simulink model "Part_2_Simulink"  (R2022b)
settings: Solver=VariableStepAuto  StartTime=0.0  StopTime=12  RelTol=1e-3
model workspace (MAT data in the model file):
  s = 351.26
  x = 425.72712
values from neighbouring files (symbols this model uses):
  Kd = PD.K    [Main.m]
  Kd_M = PD_M.K    [Main.m]
  Kd_O = PD_O.K    [Main.m]
  Kd_U = PD_U.K    [Main.m]
  Kp = -cell2mat(PD.Z)*Kd    [Main.m]
  Kp_M = -cell2mat(PD_M.Z)*Kd    [Main.m]
  Kp_O = -cell2mat(PD_O.Z)*Kd    [Main.m]
  Kp_U = -cell2mat(PD_U.Z)*Kd    [Main.m]
undefined symbols (not defined in the file or in its folder): sigbuilder_block
libraries: simulink_extras x10
settings Model: PacingRate=0.890000  Creator=AORUC19  LastModifiedBy=TANDAC20
settings OptimizationCC: ReuseModelBlockBuffer=on
settings DebuggingCC: UnconnectedInputMsg=warning  UnconnectedOutputMsg=warning  UnconnectedLineMsg=warning
settings ModelReferenceCC: EnableRefExpFcnMdlSchedulingChecks=on
settings RTWCC: DLArmComputeVersion=19.05

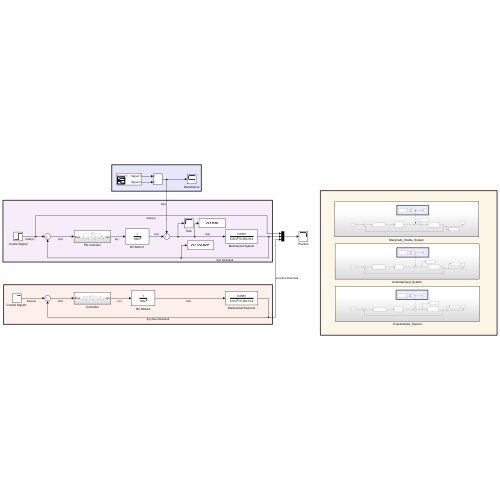
[thumbnail: Simulink's stored preview of the top-level diagram]
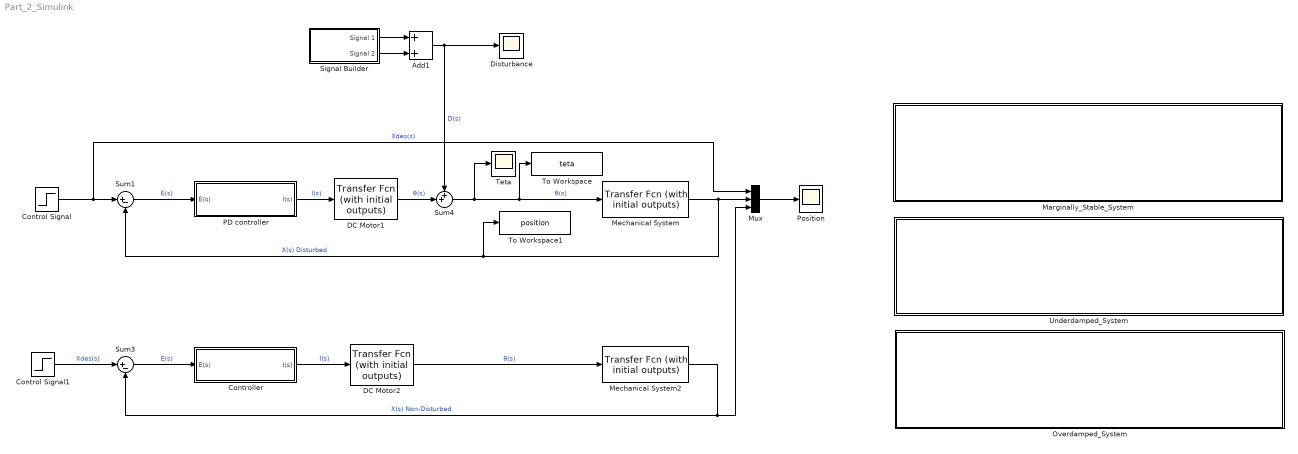
== system Part_2_Simulink ==
  Add1 : Sum
  Control Signal : Step  Time=0.3  Before=-1  After=0  SampleTime=0
  Control Signal1 : Step  Time=0.3  Before=-1  After=0  SampleTime=0
  Controller : Subsystem
  DC Motor1 : simulink_extras/Additional Linear/Transfer Fcn (with initial outputs)  N=[1]  D="[100  0 0]"  Y0=0  U0=0
  DC Motor2 : simulink_extras/Additional Linear/Transfer Fcn (with initial outputs)  N=[1]  D="[100  0 0]"  Y0=0  U0=0
  Disturbance : Scope
  Marginally_Stable_System : Subsystem
  Mechanical System : simulink_extras/Additional Linear/Transfer Fcn (with initial outputs)  N=[0.0981]  D="[0.01  0.05 0.2]"  Y0=0  U0=0
  Mechanical System2 : simulink_extras/Additional Linear/Transfer Fcn (with initial outputs)  N=[0.0981]  D="[0.01  0.05 0.2]"  Y0=0  U0=0
  Mux : Mux  Inputs=3
  Overdamped_System : Subsystem
  PD controller : Subsystem
  Position : Scope
  Signal Builder : Subsystem  Tag=STV Subsys  LoadFcn=sigbuilder_block('load');  StartFcn=sigbuilder_block('start');  StopFcn=sigbuilder_block('stop');  ClipboardFcn=sigbuilder_block('clipboard');  mask(Sigbuilder block){tuvar=[0:10]}
      mask help: Simulink:masks:SigbuilderBlock_MD
      mask init:
      | if ~strcmp(get_param(bdroot(gcbh),'SimulationStatus'),'stopped') tuvar = sigbuilder_block('maskInit'); end
      settings: CopyFcn=sigbuilder_block('copy');  DeleteFcn=sigbuilder_block('delete');  ModelCloseFcn=sigbuilder_block('modelClose');  PreSaveFcn=sigbuilder_block('preSave');  PauseFcn=sigbuilder_block('pause');  ContinueFcn=sigbuilder_block('continue');  NameChangeFcn=sigbuilder_block('namechange');  OpenFcn=sigbuilder_block('open',[437.6 199.2 550.4 400 ]);  CloseFcn=sigbuilder_block('close');
      mask Display: plot(0, 0, 100, 100,[2, 2, 32, 32, 2], [68, 8, 8, 68, 68],[32, 2], [38, 38], [32, 19, 2],[53, 60, 44], [32, 17, 17, 2],[16, 16, 31, 31]);txt = getActiveGroup(gcbh);text(2, 100, txt,'verticalAlignment', 'top');
  Sum1 : Sum  Inputs=|+-
  Sum3 : Sum  Inputs=|+-
  Sum4 : Sum  Inputs=++|
  Teta : Scope
  To Workspace : ToWorkspace  VariableName=teta  SampleTime=0.01
      settings: Save2DSignal=2-D array (concatenate along first dimension)
  To Workspace1 : ToWorkspace  VariableName=position  SampleTime=0.01
      settings: Save2DSignal=2-D array (concatenate along first dimension)
  Underdamped_System : Subsystem
  wires:
  Control Signal/1 -> Mux/1, Sum1/1  "Xdes(s)"
  Add1/1 -> Disturbance/1, Sum4/1  "D(s)"
  Signal Builder/2(Signal 2) -> Add1/2
  Signal Builder/1(Signal 1) -> Add1/1
  Mechanical System/1 -> Mux/2, To Workspace1/1, Sum1/2  "X(s) Disturbed"
  Mux/1 -> Position/1
  DC Motor2/1 -> Mechanical System2/1  "θ(s)"
  Mechanical System2/1 -> Sum3/2, Mux/3  "X(s) Non-Disturbed"
  Control Signal1/1 -> Sum3/1  "Xdes(s)"
  DC Motor1/1 -> Sum4/2  "θ(s)"
  Sum4/1 -> Mechanical System/1, To Workspace/1, Teta/1  "θ(s)"
  Sum3/1 -> Controller/1(E(s))  "E(s)"
  Controller/1(I(s)) -> DC Motor2/1  "I(s)"
  Sum1/1 -> PD controller/1(E(s))  "E(s)"
  PD controller/1(I(s)) -> DC Motor1/1  "I(s)"

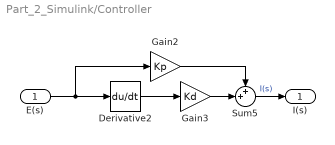
== system Part_2_Simulink/Controller ==
  E(s) : Inport
  Derivative2 : Derivative  CoefficientInTFapproximation=107.32
  Gain2 : Gain  Gain=Kp
  Gain3 : Gain  Gain=Kd
  Sum5 : Sum  Inputs=++|
  I(s) : Outport
  wires:
  Derivative2/1 -> Gain3/1
  E(s)/1 -> Derivative2/1, Gain2/1
  Gain3/1 -> Sum5/2
  Gain2/1 -> Sum5/1
  Sum5/1 -> I(s)/1  "I(s)"

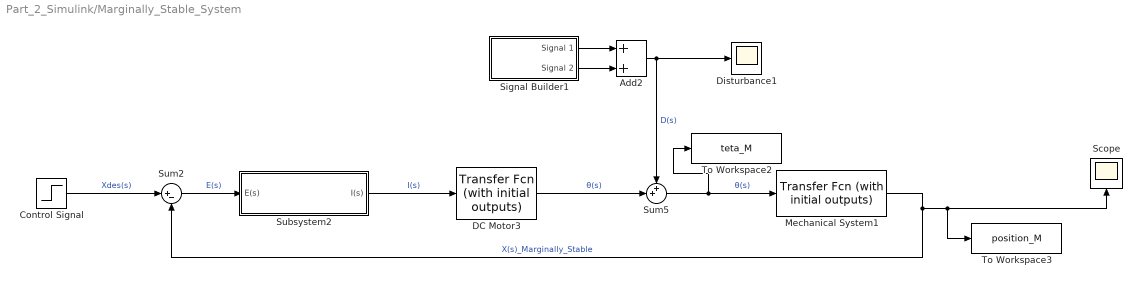
== system Part_2_Simulink/Marginally_Stable_System ==
  Add2 : Sum
  Control Signal : Step  Time=0  After=0  SampleTime=0
  DC Motor3 : simulink_extras/Additional Linear/Transfer Fcn (with initial outputs)  N=[1]  D="[100  0 0]"  Y0=0  U0=0
  Disturbance1 : Scope
  Mechanical System1 : simulink_extras/Additional Linear/Transfer Fcn (with initial outputs)  N=[0.0981]  D="[0.01  0.05 0.2]"  Y0=0  U0=0
  Scope : Scope
  Signal Builder1 : Subsystem  Tag=STV Subsys  LoadFcn=sigbuilder_block('load');  StartFcn=sigbuilder_block('start');  StopFcn=sigbuilder_block('stop');  ClipboardFcn=sigbuilder_block('clipboard');  mask(Sigbuilder block){tuvar=[0:10]}
      mask help: Simulink:masks:SigbuilderBlock_MD
      mask init:
      | if ~strcmp(get_param(bdroot(gcbh),'SimulationStatus'),'stopped') tuvar = sigbuilder_block('maskInit'); end
      settings: CopyFcn=sigbuilder_block('copy');  DeleteFcn=sigbuilder_block('delete');  ModelCloseFcn=sigbuilder_block('modelClose');  PreSaveFcn=sigbuilder_block('preSave');  PauseFcn=sigbuilder_block('pause');  ContinueFcn=sigbuilder_block('continue');  NameChangeFcn=sigbuilder_block('namechange');  OpenFcn=sigbuilder_block('open',[437.6 199.2 550.4 400 ]);  CloseFcn=sigbuilder_block('close');
      mask Display: plot(0, 0, 100, 100,[2, 2, 32, 32, 2], [68, 8, 8, 68, 68],[32, 2], [38, 38], [32, 19, 2],[53, 60, 44], [32, 17, 17, 2],[16, 16, 31, 31]);txt = getActiveGroup(gcbh);text(2, 100, txt,'verticalAlignment', 'top');
  Subsystem2 : Subsystem
  Sum2 : Sum  Inputs=|+-
  Sum5 : Sum  Inputs=++|
  To Workspace2 : ToWorkspace  VariableName=teta_M  SampleTime=0.01
      settings: Save2DSignal=2-D array (concatenate along first dimension)
  To Workspace3 : ToWorkspace  VariableName=position_M  SampleTime=0.01
      settings: Save2DSignal=2-D array (concatenate along first dimension)
  wires:
  Signal Builder1/1(Signal 1) -> Add2/1
  DC Motor3/1 -> Sum5/2  "θ(s)"
  Sum5/1 -> To Workspace2/1, Mechanical System1/1  "θ(s)"
  Signal Builder1/2(Signal 2) -> Add2/2
  Sum2/1 -> Subsystem2/1(E(s))  "E(s)"
  Mechanical System1/1 -> Scope/1, To Workspace3/1, Sum2/2  "X(s)_Marginally_Stable"
  Subsystem2/1(I(s)) -> DC Motor3/1  "I(s)"
  Add2/1 -> Disturbance1/1, Sum5/1  "D(s)"
  Control Signal/1 -> Sum2/1  "Xdes(s)"

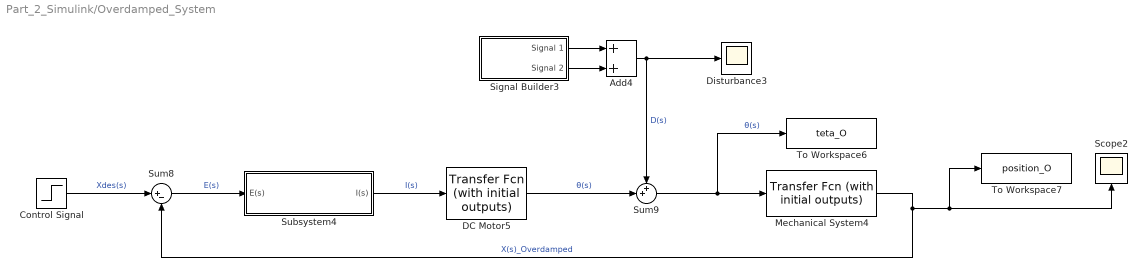
== system Part_2_Simulink/Overdamped_System ==
  Add4 : Sum
  Control Signal : Step  Time=0  After=0  SampleTime=0
  DC Motor5 : simulink_extras/Additional Linear/Transfer Fcn (with initial outputs)  N=[1]  D="[100  0 0]"  Y0=0  U0=0
  Disturbance3 : Scope
  Mechanical System4 : simulink_extras/Additional Linear/Transfer Fcn (with initial outputs)  N=[0.0981]  D="[0.01  0.05 0.2]"  Y0=0  U0=0
  Scope2 : Scope
  Signal Builder3 : Subsystem  Tag=STV Subsys  LoadFcn=sigbuilder_block('load');  StartFcn=sigbuilder_block('start');  StopFcn=sigbuilder_block('stop');  ClipboardFcn=sigbuilder_block('clipboard');  mask(Sigbuilder block){tuvar=[0:10]}
      mask help: Simulink:masks:SigbuilderBlock_MD
      mask init:
      | if ~strcmp(get_param(bdroot(gcbh),'SimulationStatus'),'stopped') tuvar = sigbuilder_block('maskInit'); end
      settings: CopyFcn=sigbuilder_block('copy');  DeleteFcn=sigbuilder_block('delete');  ModelCloseFcn=sigbuilder_block('modelClose');  PreSaveFcn=sigbuilder_block('preSave');  PauseFcn=sigbuilder_block('pause');  ContinueFcn=sigbuilder_block('continue');  NameChangeFcn=sigbuilder_block('namechange');  OpenFcn=sigbuilder_block('open',[437.6 199.2 550.4 400 ]);  CloseFcn=sigbuilder_block('close');
      mask Display: plot(0, 0, 100, 100,[2, 2, 32, 32, 2], [68, 8, 8, 68, 68],[32, 2], [38, 38], [32, 19, 2],[53, 60, 44], [32, 17, 17, 2],[16, 16, 31, 31]);txt = getActiveGroup(gcbh);text(2, 100, txt,'verticalAlignment', 'top');
  Subsystem4 : Subsystem
  Sum8 : Sum  Inputs=|+-
  Sum9 : Sum  Inputs=++|
  To Workspace6 : ToWorkspace  VariableName=teta_O  SampleTime=0.01
      settings: Save2DSignal=2-D array (concatenate along first dimension)
  To Workspace7 : ToWorkspace  VariableName=position_O  SampleTime=0.01
      settings: Save2DSignal=2-D array (concatenate along first dimension)
  wires:
  Add4/1 -> Disturbance3/1, Sum9/1  "D(s)"
  Signal Builder3/2(Signal 2) -> Add4/2
  Sum8/1 -> Subsystem4/1(E(s))  "E(s)"
  Mechanical System4/1 -> To Workspace7/1, Scope2/1, Sum8/2  "X(s)_Overdamped"
  Sum9/1 -> To Workspace6/1, Mechanical System4/1  "θ(s)"
  Signal Builder3/1(Signal 1) -> Add4/1
  DC Motor5/1 -> Sum9/2  "θ(s)"
  Subsystem4/1(I(s)) -> DC Motor5/1  "I(s)"
  Control Signal/1 -> Sum8/1  "Xdes(s)"

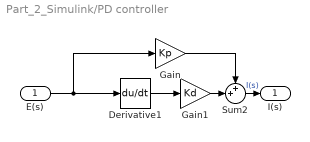
== system Part_2_Simulink/PD controller ==
  E(s) : Inport
  Derivative1 : Derivative  CoefficientInTFapproximation=107.32
  Gain : Gain  Gain=Kp
  Gain1 : Gain  Gain=Kd
  Sum2 : Sum  Inputs=++|
  I(s) : Outport
  wires:
  Gain/1 -> Sum2/1
  Derivative1/1 -> Gain1/1
  Gain1/1 -> Sum2/2
  Sum2/1 -> I(s)/1  "I(s)"
  E(s)/1 -> Gain/1, Derivative1/1

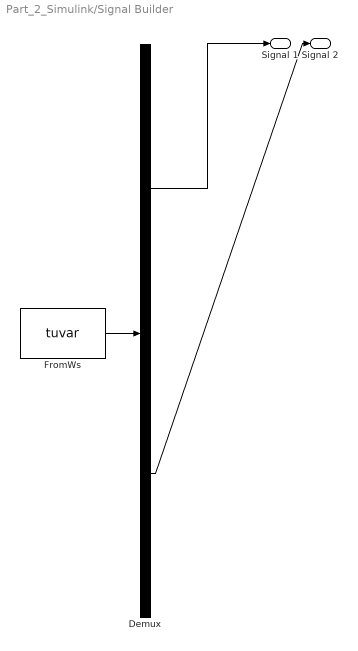
== system Part_2_Simulink/Signal Builder ==
  Demux : Demux  Tag=STV Demux  Outputs=2
      settings: DisplayOption=none
  FromWs : FromWorkspace  Tag=STV FromWs  VariableName=tuvar
      SigBuilderData=|
      | common.afterFinalStr = 'Extrapolate'
      | common.sampleTime = 0
      | dataSet.timeRange = [0 10]
      | dataSet.name = 'Group 1'
      | sbobj.Groups.Name = 'Group 1'
      | sbobj.Groups.Signals(1).Name = 'Signal 1'
      | sbobj.Groups.Signals(1).XData = [0 2 2 2.1 2.1 10]
      | sbobj.Groups.Signals(1).YData = [0 0 0.52 0.52 0 0]
      | sbobj.Groups.Signals(2).Name = 'Signal 2'
      | sbobj.Groups.Signals(2).XData = [0 6 6 8 9 10]
      | sbobj.Groups.Signals(2).YData = [0 0 -0.52 0 0 0]
  Signal 1 : Outport  Tag=STV Outport
  Signal 2 : Outport  Tag=STV Outport  Port=2
  wires:
  Demux/2 -> Signal 2/1
  FromWs/1 -> Demux/1
  Demux/1 -> Signal 1/1

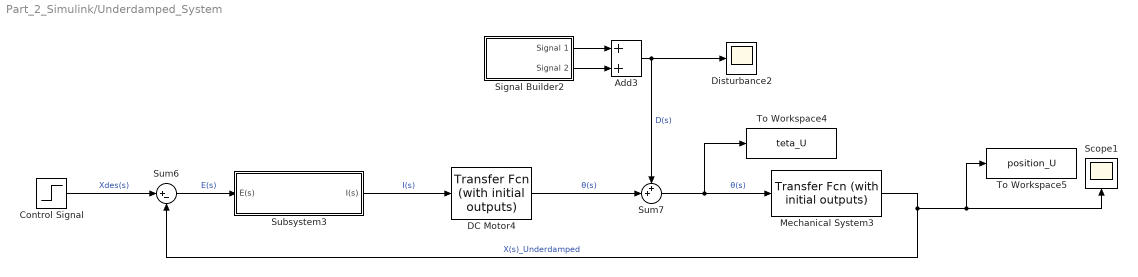
== system Part_2_Simulink/Underdamped_System ==
  Add3 : Sum
  Control Signal : Step  Time=0  After=0  SampleTime=0
  DC Motor4 : simulink_extras/Additional Linear/Transfer Fcn (with initial outputs)  N=[1]  D="[100  0 0]"  Y0=0  U0=0
  Disturbance2 : Scope
  Mechanical System3 : simulink_extras/Additional Linear/Transfer Fcn (with initial outputs)  N=[0.0981]  D="[0.01  0.05 0.2]"  Y0=0  U0=0
  Scope1 : Scope
  Signal Builder2 : Subsystem  Tag=STV Subsys  LoadFcn=sigbuilder_block('load');  StartFcn=sigbuilder_block('start');  StopFcn=sigbuilder_block('stop');  ClipboardFcn=sigbuilder_block('clipboard');  mask(Sigbuilder block){tuvar=[0:10]}
      mask help: Simulink:masks:SigbuilderBlock_MD
      mask init:
      | if ~strcmp(get_param(bdroot(gcbh),'SimulationStatus'),'stopped') tuvar = sigbuilder_block('maskInit'); end
      settings: CopyFcn=sigbuilder_block('copy');  DeleteFcn=sigbuilder_block('delete');  ModelCloseFcn=sigbuilder_block('modelClose');  PreSaveFcn=sigbuilder_block('preSave');  PauseFcn=sigbuilder_block('pause');  ContinueFcn=sigbuilder_block('continue');  NameChangeFcn=sigbuilder_block('namechange');  OpenFcn=sigbuilder_block('open',[437.6 199.2 550.4 400 ]);  CloseFcn=sigbuilder_block('close');
      mask Display: plot(0, 0, 100, 100,[2, 2, 32, 32, 2], [68, 8, 8, 68, 68],[32, 2], [38, 38], [32, 19, 2],[53, 60, 44], [32, 17, 17, 2],[16, 16, 31, 31]);txt = getActiveGroup(gcbh);text(2, 100, txt,'verticalAlignment', 'top');
  Subsystem3 : Subsystem
  Sum6 : Sum  Inputs=|+-
  Sum7 : Sum  Inputs=++|
  To Workspace4 : ToWorkspace  VariableName=teta_U  SampleTime=0.01
      settings: Save2DSignal=2-D array (concatenate along first dimension)
  To Workspace5 : ToWorkspace  VariableName=position_U  SampleTime=0.01
      settings: Save2DSignal=2-D array (concatenate along first dimension)
  wires:
  Sum7/1 -> To Workspace4/1, Mechanical System3/1  "θ(s)"
  Subsystem3/1(I(s)) -> DC Motor4/1  "I(s)"
  Mechanical System3/1 -> To Workspace5/1, Scope1/1, Sum6/2  "X(s)_Underdamped"
  Signal Builder2/2(Signal 2) -> Add3/2
  DC Motor4/1 -> Sum7/2  "θ(s)"
  Add3/1 -> Disturbance2/1, Sum7/1  "D(s)"
  Sum6/1 -> Subsystem3/1(E(s))  "E(s)"
  Signal Builder2/1(Signal 1) -> Add3/1
  Control Signal/1 -> Sum6/1  "Xdes(s)"

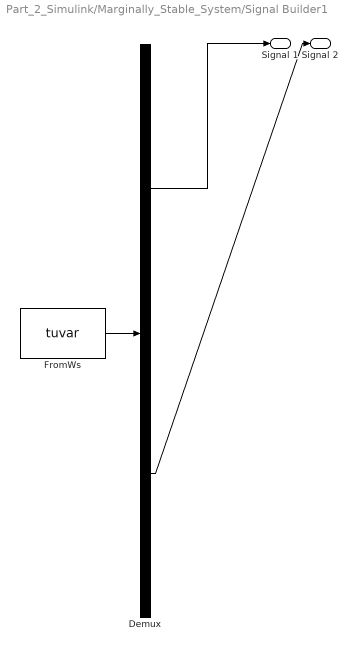
== system Part_2_Simulink/Marginally_Stable_System/Signal Builder1 ==
  Demux : Demux  Tag=STV Demux  Outputs=2
      settings: DisplayOption=none
  FromWs : FromWorkspace  Tag=STV FromWs  VariableName=tuvar
      SigBuilderData=|
      | common.afterFinalStr = 'Extrapolate'
      | common.sampleTime = 0
      | dataSet.timeRange = [0 10]
      | dataSet.name = 'Group 1'
      | sbobj.Groups.Name = 'Group 1'
      | sbobj.Groups.Signals(1).Name = 'Signal 1'
      | sbobj.Groups.Signals(1).XData = [0 2 2 2.1 2.1 10]
      | sbobj.Groups.Signals(1).YData = [0 0 0.52 0.52 0 0]
      | sbobj.Groups.Signals(2).Name = 'Signal 2'
      | sbobj.Groups.Signals(2).XData = [0 6 6 8 9 10]
      | sbobj.Groups.Signals(2).YData = [0 0 -0.52 0 0 0]
  Signal 1 : Outport  Tag=STV Outport
  Signal 2 : Outport  Tag=STV Outport  Port=2
  wires:
  Demux/2 -> Signal 2/1
  FromWs/1 -> Demux/1
  Demux/1 -> Signal 1/1

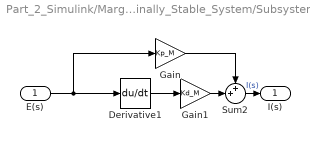
== system Part_2_Simulink/Marginally_Stable_System/Subsystem2 ==
  E(s) : Inport
  Derivative1 : Derivative  CoefficientInTFapproximation=107.32
  Gain : Gain  Gain=Kp_M
  Gain1 : Gain  Gain=Kd_M
  Sum2 : Sum  Inputs=++|
  I(s) : Outport
  wires:
  Gain/1 -> Sum2/1
  Derivative1/1 -> Gain1/1
  Gain1/1 -> Sum2/2
  Sum2/1 -> I(s)/1  "I(s)"
  E(s)/1 -> Gain/1, Derivative1/1

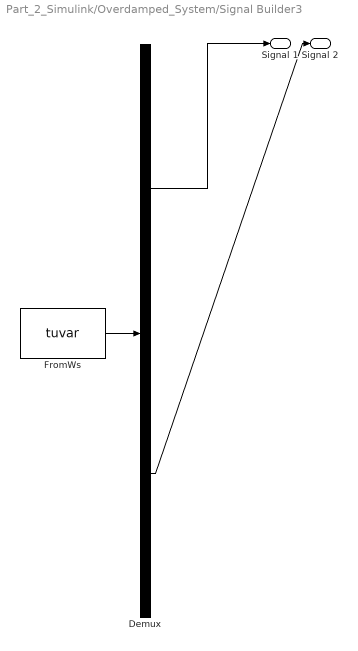
== system Part_2_Simulink/Overdamped_System/Signal Builder3 ==
  Demux : Demux  Tag=STV Demux  Outputs=2
      settings: DisplayOption=none
  FromWs : FromWorkspace  Tag=STV FromWs  VariableName=tuvar
      SigBuilderData=|
      | common.afterFinalStr = 'Extrapolate'
      | common.sampleTime = 0
      | dataSet.timeRange = [0 10]
      | dataSet.name = 'Group 1'
      | sbobj.Groups.Name = 'Group 1'
      | sbobj.Groups.Signals(1).Name = 'Signal 1'
      | sbobj.Groups.Signals(1).XData = [0 2 2 2.1 2.1 10]
      | sbobj.Groups.Signals(1).YData = [0 0 0.52 0.52 0 0]
      | sbobj.Groups.Signals(2).Name = 'Signal 2'
      | sbobj.Groups.Signals(2).XData = [0 6 6 8 9 10]
      | sbobj.Groups.Signals(2).YData = [0 0 -0.52 0 0 0]
  Signal 1 : Outport  Tag=STV Outport
  Signal 2 : Outport  Tag=STV Outport  Port=2
  wires:
  Demux/2 -> Signal 2/1
  FromWs/1 -> Demux/1
  Demux/1 -> Signal 1/1

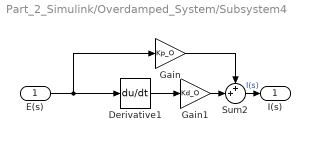
== system Part_2_Simulink/Overdamped_System/Subsystem4 ==
  E(s) : Inport
  Derivative1 : Derivative  CoefficientInTFapproximation=107.32
  Gain : Gain  Gain=Kp_O
  Gain1 : Gain  Gain=Kd_O
  Sum2 : Sum  Inputs=++|
  I(s) : Outport
  wires:
  Gain/1 -> Sum2/1
  Derivative1/1 -> Gain1/1
  Gain1/1 -> Sum2/2
  Sum2/1 -> I(s)/1  "I(s)"
  E(s)/1 -> Gain/1, Derivative1/1

== system Part_2_Simulink/Underdamped_System/Signal Builder2 ==
  Demux : Demux  Tag=STV Demux  Outputs=2
      settings: DisplayOption=none
  FromWs : FromWorkspace  Tag=STV FromWs  VariableName=tuvar
      SigBuilderData=|
      | common.afterFinalStr = 'Extrapolate'
      | common.sampleTime = 0
      | dataSet.timeRange = [0 10]
      | dataSet.name = 'Group 1'
      | sbobj.Groups.Name = 'Group 1'
      | sbobj.Groups.Signals(1).Name = 'Signal 1'
      | sbobj.Groups.Signals(1).XData = [0 2 2 2.1 2.1 10]
      | sbobj.Groups.Signals(1).YData = [0 0 0.52 0.52 0 0]
      | sbobj.Groups.Signals(2).Name = 'Signal 2'
      | sbobj.Groups.Signals(2).XData = [0 6 6 8 9 10]
      | sbobj.Groups.Signals(2).YData = [0 0 -0.52 0 0 0]
  Signal 1 : Outport  Tag=STV Outport
  Signal 2 : Outport  Tag=STV Outport  Port=2
  wires:
  Demux/2 -> Signal 2/1
  FromWs/1 -> Demux/1
  Demux/1 -> Signal 1/1

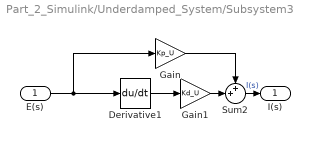
== system Part_2_Simulink/Underdamped_System/Subsystem3 ==
  E(s) : Inport
  Derivative1 : Derivative  CoefficientInTFapproximation=107.32
  Gain : Gain  Gain=Kp_U
  Gain1 : Gain  Gain=Kd_U
  Sum2 : Sum  Inputs=++|
  I(s) : Outport
  wires:
  Gain/1 -> Sum2/1
  Derivative1/1 -> Gain1/1
  Gain1/1 -> Sum2/2
  Sum2/1 -> I(s)/1  "I(s)"
  E(s)/1 -> Gain/1, Derivative1/1
